simulink model "coolingskid_digitaltwin"  (R2026a)
settings: Solver=VariableStepAuto  StopTime=600
libraries: fl_lib x12, nesl_utility x7, SimscapeFluids_lib x1
settings Model: Creator=novik  LastModifiedBy=novik

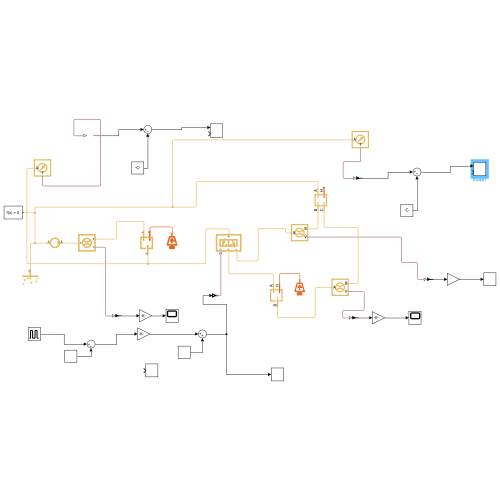
[thumbnail: Simulink's stored preview of the top-level diagram]
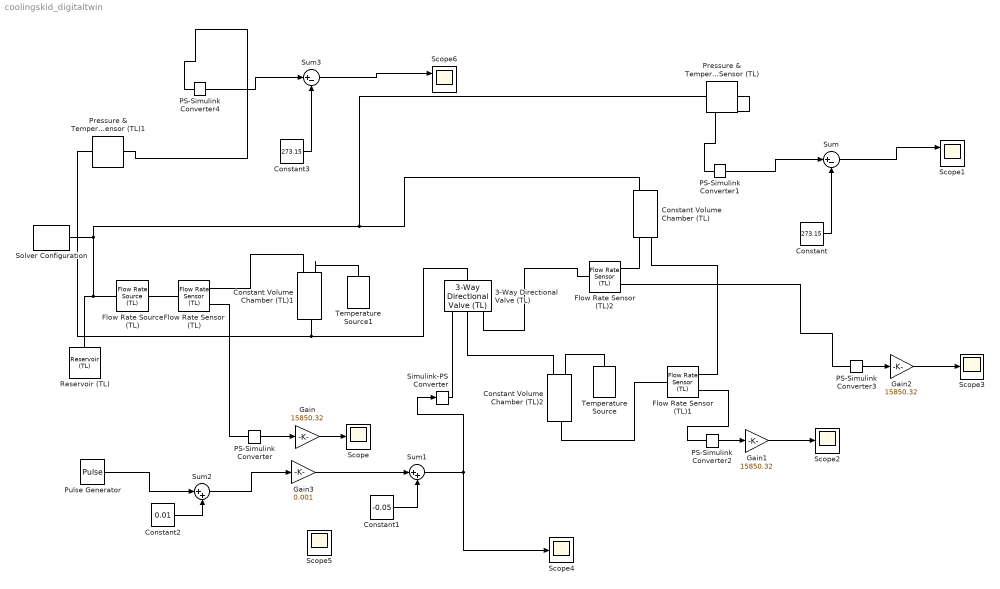
== system coolingskid_digitaltwin ==
  3-Way Directional Valve (TL) : SimscapeFluids_lib/Thermal Liquid/Valves & Orifices/Directional Control Valves/3-Way Directional Valve (TL)  open_orifices_pos=fluids.thermal_liquid.valves.directional_control_valves.enum.OpenOrifices3Way.PA  open_orifices_neg=fluids.thermal_liquid.valves.directional_control_valves.enum.OpenOrifices3Way.AT  area_spec=fluids.thermal_liquid.valves.directional_control_valves.enum.area_spec.identical  valve_spec=fluids.thermal_liquid.valves.directional_control_valves.enum.ValveSpec.Linear  del_S_max=.1 m  area_max=.165 in^2  del_S_TLU=[0, .00125, .0025, .00375, .005] m  valve_area_TLU=[1e-10, 1e-05, 4e-05, 8e-05, .0001] m^2  del_S_flow_TLU=[0, .00125, .0025, .00375, .005] m  p_diff_TLU=[-.1, .3, .5, .7] MPa  vol_flow_TLU=[-9.05e-10, 1.57e-09, 2.02e-09, 2.39e-09; -9.05e-05, .000157, .000202, .000239; -.000362, .000627, .00081, .000958; -.000724, .00125, .00162, .00192; -.000905, .00156, .002, .00239] gpm  mdot_TLU=1e3 * [-9.05e-10, 1.57e-09, 2.02e-09, 2.39e-09; -9.05e-05, .000157, .000202, .000239; -.000362, .000627, .00081, .000958; -.000724, .00125, .00162, .00192; -.000905, .00156, .002, .00239] kg/s  T_ref_in=293.15 K  p_ref_in=0.101325 MPa  area_leak=1e-10 m^2  Cd=0.64  Re_c=150  smoothing_factor=0.01  pressure_recovery=false  area=.17 in^2  S_max_PA=.05 m  del_S_max_PA=0.005 m  area_max_PA=1e-4 m^2  del_S_TLU_PA=[0, .00125, .0025, .00375, .005] m  valve_area_TLU_PA=[1e-10, 1e-05, 4e-05, 8e-05, .0001] m^2  del_S_flow_TLU_PA=[0, .00125, .0025, .00375, .005] m  p_diff_TLU_PA=[-.1, .3, .5, .7] MPa  vol_flow_TLU_PA=[-9.05e-10, 1.57e-09, 2.02e-09, 2.39e-09; -9.05e-05, .000157, .000202, .000239; -.000362, .000627, .00081, .000958; -.000724, .00125, .00162, .00192; -.000905, .00156, .002, .00239] m^3/s  mdot_TLU_PA=1e3 * [-9.05e-10, 1.57e-09, 2.02e-09, 2.39e-09; -9.05e-05, .000157, .000202, .000239; -.000362, .000627, .00081, .000958; -.000724, .00125, .00162, .00192; -.000905, .00156, .002, .00239] kg/s  S_max_AT=-.05 m  del_S_max_AT=0.005 m  area_max_AT=1e-4 m^2  del_S_TLU_AT=[0, .00125, .0025, .00375, .005] m  valve_area_TLU_AT=[1e-10, 1e-05, 4e-05, 8e-05, .0001] m^2  del_S_flow_TLU_AT=[0, .00125, .0025, .00375, .005] m  p_diff_TLU_AT=[-.1, .3, .5, .7] MPa  vol_flow_TLU_AT=[-9.05e-10, 1.57e-09, 2.02e-09, 2.39e-09; -9.05e-05, .000157, .000202, .000239; -.000362, .000627, .00081, .000958; -.000724, .00125, .00162, .00192; -.000905, .00156, .002, .00239] m^3/s  mdot_TLU_AT=1e3 * [-9.05e-10, 1.57e-09, 2.02e-09, 2.39e-09; -9.05e-05, .000157, .000202, .000239; -.000362, .000627, .00081, .000958; -.000724, .00125, .00162, .00192; -.000905, .00156, .002, .00239] kg/s  S_max_PT=4.5e-3 m  del_S_max_PT=0.005 m  area_max_PT=1e-4 m^2  del_S_TLU_PT=[0, .00125, .0025, .00375, .005] m  valve_area_TLU_PT=[1e-10, 1e-05, 4e-05, 8e-05, .0001] m^2  del_S_flow_TLU_PT=[0, .00125, .0025, .00375, .005] m  p_diff_TLU_PT=[-.1, .3, .5, .7] MPa  vol_flow_TLU_PT=[-9.05e-10, 1.57e-09, 2.02e-09, 2.39e-09; -9.05e-05, .000157, .000202, .000239; -.000362, .000627, .00081, .000958; -.000724, .00125, .00162, .00192; -.000905, .00156, .002, .00239] m^3/s  mdot_TLU_PT=1e3 * [-9.05e-10, 1.57e-09, 2.02e-09, 2.39e-09; -9.05e-05, .000157, .000202, .000239; -.000362, .000627, .00081, .000958; -.000724, .00125, .00162, .00192; -.000905, .00156, .002, .00239] kg/s
  Constant : Constant  Value=273.15
  Constant Volume Chamber (TL) : fl_lib/Thermal Liquid/Elements/Constant Volume Chamber (TL)  volume=0.05 gal  num_ports=foundation.enum.num_ports.three  area_A=0.17 in^2  area_B=0.17 in^2  area_C=0.17 in^2  area_D=0.01 m^2  p_I_specify=off  p_I_priority=High  p_I=0.101325 MPa  p_I_nominal_specify=off  p_I_nominal_value=1  p_I_nominal_unit=MPa  T_I_specify=on  T_I_priority=High  T_I=35 degC  T_I_nominal_specify=off  T_I_nominal_value=35  T_I_nominal_unit=degC  u_I_specify=off  u_I_priority=None  u_I=83.906 kJ/kg  u_I_nominal_specify=off  u_I_nominal_value=1  u_I_nominal_unit=kJ/kg  rho_I_specify=off  rho_I_priority=None  rho_I=998.21 kg/m^3  rho_I_nominal_specify=off  rho_I_nominal_value=1  rho_I_nominal_unit=kg/m^3
  Constant Volume Chamber (TL)1 : fl_lib/Thermal Liquid/Elements/Constant Volume Chamber (TL)  volume=4 gal  num_ports=foundation.enum.num_ports.two  area_A=0.17 in^2  area_B=0.17 in^2  area_C=0.17 in^2  area_D=0.01 m^2  p_I_specify=off  p_I_priority=High  p_I=0.101325 MPa  p_I_nominal_specify=off  p_I_nominal_value=1  p_I_nominal_unit=MPa  T_I_specify=on  T_I_priority=High  T_I=35 degC  T_I_nominal_specify=off  T_I_nominal_value=35  T_I_nominal_unit=degC  u_I_specify=off  u_I_priority=None  u_I=83.906 kJ/kg  u_I_nominal_specify=off  u_I_nominal_value=1  u_I_nominal_unit=kJ/kg  rho_I_specify=off  rho_I_priority=None  rho_I=998.21 kg/m^3  rho_I_nominal_specify=off  rho_I_nominal_value=1  rho_I_nominal_unit=kg/m^3
  Constant Volume Chamber (TL)2 : fl_lib/Thermal Liquid/Elements/Constant Volume Chamber (TL)  volume=4 gal  num_ports=foundation.enum.num_ports.two  area_A=0.17 in^2  area_B=0.17 in^2  area_C=0.17 in^2  area_D=0.01 m^2  p_I_specify=off  p_I_priority=High  p_I=0.101325 MPa  p_I_nominal_specify=off  p_I_nominal_value=1  p_I_nominal_unit=MPa  T_I_specify=on  T_I_priority=High  T_I=35 degC  T_I_nominal_specify=off  T_I_nominal_value=35  T_I_nominal_unit=degC  u_I_specify=off  u_I_priority=None  u_I=83.906 kJ/kg  u_I_nominal_specify=off  u_I_nominal_value=1  u_I_nominal_unit=kJ/kg  rho_I_specify=off  rho_I_priority=None  rho_I=998.21 kg/m^3  rho_I_nominal_specify=off  rho_I_nominal_value=1  rho_I_nominal_unit=kg/m^3
  Constant1 : Constant  Value=-0.05
  Constant2 : Constant  Value=0.01
  Constant3 : Constant  Value=273.15
  Flow Rate Sensor (TL) : fl_lib/Thermal Liquid/Sensors/Flow Rate Sensor (TL)  mass_flow_measure=false  volumetric_flow_measure=true  energy_flow_measure=false
  Flow Rate Sensor (TL)1 : fl_lib/Thermal Liquid/Sensors/Flow Rate Sensor (TL)  mass_flow_measure=false  volumetric_flow_measure=true  energy_flow_measure=false
  Flow Rate Sensor (TL)2 : fl_lib/Thermal Liquid/Sensors/Flow Rate Sensor (TL)  mass_flow_measure=false  volumetric_flow_measure=true  energy_flow_measure=false
  Flow Rate Source (TL) : fl_lib/Thermal Liquid/Sources/Flow Rate Source (TL)  source_type=foundation.enum.constant_controlled.constant  flow_type=foundation.enum.mass_volumetric_flow.volumetric  mass_flow=0 kg/s  volumetric_flow=.35 gpm  power_spec=foundation.enum.power_spec.none  area=.17 in^2
  Gain : Gain  Gain=15850.32
  Gain1 : Gain  Gain=15850.32
  Gain2 : Gain  Gain=15850.32
  Gain3 : Gain  Gain=0.001
  PS-Simulink Converter{,1..4} (5 alike) : nesl_utility/PS-Simulink Converter  PhysicalDomain=network_engine_domain  SubClassName=ps_output  LeftPortType=input  RightPortType=output  PseudoPeriodic=off  Frequencies=[]  VectorFormat=inherit  Unit=inherit  AffineConversion=off
  Pressure & Temperature Sensor (TL) : fl_lib/Thermal Liquid/Sensors/Pressure & Temperature Sensor (TL)  reference=foundation.enum.MeasurementReference.absolute  pressure=false  pressure_spec=foundation.enum.PressureMeasementSpec.Absolute  temperature=true
  Pressure & Temperature Sensor (TL)1 : fl_lib/Thermal Liquid/Sensors/Pressure & Temperature Sensor (TL)  reference=foundation.enum.MeasurementReference.absolute  pressure=false  pressure_spec=foundation.enum.PressureMeasementSpec.Absolute  temperature=true
  Pulse Generator : DiscretePulseGenerator  PulseType=Time based  Amplitude=99.9  Period=150  PulseWidth=95
  Reservoir (TL) : fl_lib/Thermal Liquid/Elements/Reservoir (TL)  pressure_input=false  pressure_spec=foundation.enum.pressure_spec.atmospheric  reservoir_pressure=0.101325 MPa  temperature_input=false  reservoir_temperature=35 degC  area=0.17 in^2  input_error_spec=foundation.enum.input_range_error.warn
  Scope{,2..5} (5 alike) : Scope
      Scope settings: ActiveDisplayYMinimum=0.34568079722781964  ActiveDisplayYMaximum=0.35008156241954713
      Scope2 settings: ActiveDisplayYMinimum=-0.10454658555824214  ActiveDisplayYMaximum=0.38855847141742039  DataLoggingVariableName=ScopeData2
      Scope3 settings: ActiveDisplayYMinimum=-0.38550745650445867  ActiveDisplayYMaximum=0.62985852793836439  DataLoggingVariableName=ScopeData3
      Scope4 settings: ActiveDisplayYMinimum=-0.094062180201090126  ActiveDisplayYMaximum=0.23697520285744753  DataLoggingVariableName=ScopeData4
      Scope5 settings: ActiveDisplayYMinimum=-57.765102675932  ActiveDisplayYMaximum=118.21100683348861  DataLoggingVariableName=ScopeData5
  Scope1 : Scope  NumInputPorts=2
      settings: ActiveDisplayYMinimum=34.453110500556747  ActiveDisplayYMaximum=39.3100155700768
  Scope6 : Scope  NumInputPorts=2
      settings: ActiveDisplayYMinimum=-73.296828165375445  ActiveDisplayYMaximum=199.02921061162277  DataLoggingVariableName=ScopeData6
  Simulink-PS Converter : nesl_utility/Simulink-PS Converter  PhysicalDomain=network_engine_domain  SubClassName=ps_input  LeftPortType=input  RightPortType=output  PseudoPeriodic=off  Frequencies=[]  NoiseDistribution=none  NoiseParameters=[]  Unit=1  AffineConversion=off  FilteringAndDerivatives=provide  SimscapeFilterOrder=1  InputFilterTimeConstant=0.001  UdotUserProvided=0
  Solver Configuration : nesl_utility/Solver Configuration  PhysicalDomain=network_engine_domain  SubClassName=solver  LeftPortType=input  RightPortType=generic  Tones=[]  Harmonics=[]  SimulateNoise=off  Profile=off  UseLocalSampling=off  EnableSwitchedLinearOptims=on  FrequencyDomain=off  UseCCode=off  RelTol=0.001  AbsTol=0.001  MinStep=1e-09  ToWorkspace=off  RevertToSquareIcSolve=off  NumHomotopyIterations=100  PhasorMode=off  PhasorModeNumHarmonics=1  ConsistencySolver=NEWTON_XTOL_AFTER_FTOL  CanonicalOrdering=CANONICAL  OptimizeIntermediates=OPTIMIZED  IndexReductionMethod=DerivativeReplacement  DoDC=off  ResidualTolerance=1e-09  ConsistencyTolSource=GLOBAL  ConsistencyAbsTol=0.001  ConsistencyRelTol=0.001  ConsistencyTolFactor=0.001  UseLocalSolver=off  LocalSolverChoice=NE_BACKWARD_EULER_ADVANCER  ResolveIndetEquations=on  FunctionEvalNumThread=1  LocalSolverSampleTime=0.001  DoFixedCost=off  MaxNonlinIter=3  MaxModeIter=2  ComputeImpulses=off  ImpulseIterations=2  LinearAlgebra=auto  LinearAlgebraNumThread=0  EquationFormulation=NE_TIME_EF  DelaysMemoryBudget=1024  AutomaticFiltering=on  FilteringTimeConstant=0.001  PartitionStorageMethod=AS_NEEDED  PartitionMemoryBudget=1024  PartitionMethod=ROBUST  MultibodyUseLocalSolver=off  MultibodyLocalSolverChoice=ODE1  MultibodyLocalSolverSampleTime=0.001
  Sum : Sum  Inputs=|+-
  Sum1 : Sum  Inputs=|++
  Sum2 : Sum  Inputs=|++
  Sum3 : Sum  Inputs=|+-
  Temperature Source : fl_lib/Thermal/Thermal Sources/Temperature Source  temperature=35 degC
  Temperature Source1 : fl_lib/Thermal/Thermal Sources/Temperature Source  temperature=41 degC
  wires:
  PS-Simulink Converter/1 -> Gain/1
  Gain/1 -> Scope/1
  PS-Simulink Converter1/1 -> Sum/1
  Constant/1 -> Sum/2
  Sum/1 -> Scope1/1
  Gain1/1 -> Scope2/1
  PS-Simulink Converter2/1 -> Gain1/1
  Gain2/1 -> Scope3/1
  PS-Simulink Converter3/1 -> Gain2/1
  Sum1/1 -> Scope4/1, Simulink-PS Converter/1
  Constant1/1 -> Sum1/2
  Gain3/1 -> Sum1/1
  Sum3/1 -> Scope6/1
  PS-Simulink Converter4/1 -> Sum3/1
  Constant3/1 -> Sum3/2
  Constant2/1 -> Sum2/2
  Pulse Generator/1 -> Sum2/1
  Sum2/1 -> Gain3/1
  connections:
  Solver Configuration/RConn1 -- Constant Volume Chamber (TL)/LConn1 -- Pressure & Temperature Sensor (TL)/LConn1 -- Flow Rate Source (TL)/LConn1 -- Reservoir (TL)/LConn1
  Flow Rate Sensor (TL)/RConn2 -- PS-Simulink Converter/LConn1
  Pressure & Temperature Sensor (TL)/RConn1 -- PS-Simulink Converter1/LConn1
  Constant Volume Chamber (TL)1/LConn1 -- Flow Rate Sensor (TL)/RConn1
  Flow Rate Sensor (TL)/LConn1 -- Flow Rate Source (TL)/RConn1
  Constant Volume Chamber (TL)1/RConn1 -- 3-Way Directional Valve (TL)/LConn1 -- Pressure & Temperature Sensor (TL)1/LConn1
  3-Way Directional Valve (TL)/RConn1 -- Simulink-PS Converter/RConn1
  PS-Simulink Converter2/LConn1 -- Flow Rate Sensor (TL)1/RConn2
  PS-Simulink Converter3/LConn1 -- Flow Rate Sensor (TL)2/RConn2
  3-Way Directional Valve (TL)/RConn3 -- Flow Rate Sensor (TL)2/LConn1
  Constant Volume Chamber (TL)2/RConn1 -- Flow Rate Sensor (TL)1/LConn1
  Constant Volume Chamber (TL)2/LConn1 -- 3-Way Directional Valve (TL)/RConn2
  Pressure & Temperature Sensor (TL)1/RConn1 -- PS-Simulink Converter4/LConn1
  Constant Volume Chamber (TL)1/LConn2 -- Temperature Source1/LConn1
  Flow Rate Sensor (TL)2/RConn1 -- Constant Volume Chamber (TL)/RConn1
  Flow Rate Sensor (TL)1/RConn1 -- Constant Volume Chamber (TL)/RConn2
  Constant Volume Chamber (TL)2/LConn2 -- Temperature Source/LConn1
